simulink model "Discrete_LADRC_Control_Simulation"  (R2025a)
settings: Solver=VariableStepAuto  StartTime=0.0  StopTime=0.3  RelTol=1e-3
libraries: powerlib_extras x1
settings Model: Creator=星必尘Sguan  LastModifiedBy=星必尘Sguan
settings SFSimCC: SimCustomHeaderCode="#include \"Sguan_Ladrc.h\""  SimCustomInitializer=Sguan_Init();  SimUserSources=Sguan_Ladrc.c

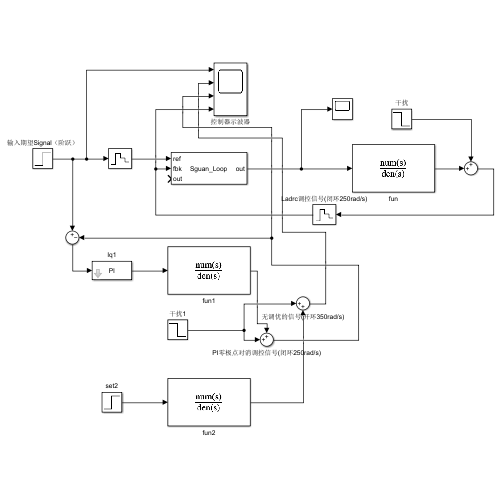
[thumbnail: Simulink's stored preview of the top-level diagram]
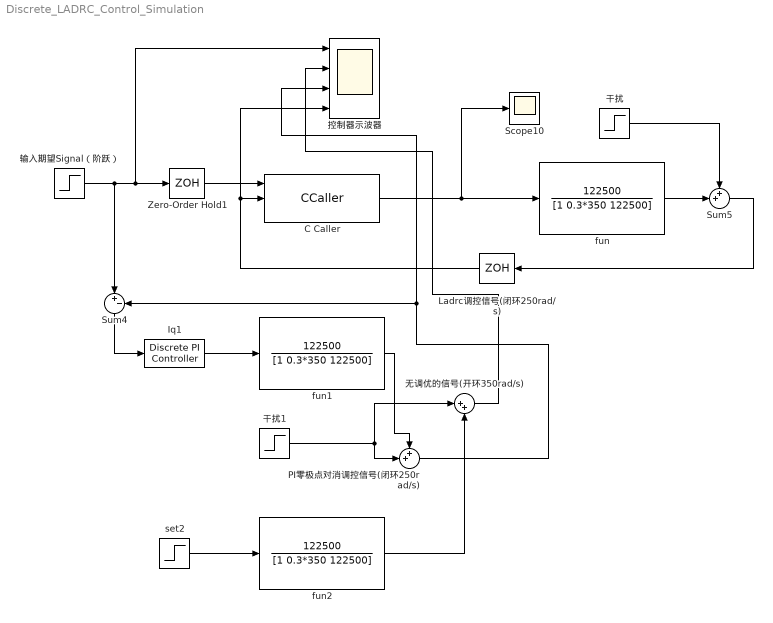
== system Discrete_LADRC_Control_Simulation ==
  C Caller : CCaller  FunctionName=Sguan_Loop  PortSpecificationStruct="%)30     .    8 4   8    (     @         %    \"     ,    !     0         %  0 \"0    $    _    07)G3F%M90  4&]R=$YA;64 4V-O<&4     26YD97@     5'EP90      4VEZ90      27-';&]B86P   X    P    !@    @    $          4    (     0    ,    !         !   P!R968 #@   #     &    \"     0         !0    @    !     P    $         $  # ')E9@ .    .     8    (    !          %    \"     $    %     0         0    !0   $EN<'5T    #@   #@    &    \"     8         !0    @    !     0    $         \"0    @               X    X    !@    @    $          4    (     0    8    !         !     &    9&]U8FQE   .    ,     8    (    !          %    \"     $    !     0         0  $ ,0    X    P    !@    @    ) @        4    (     0    $    !          (  0      #@   #     &    \"     0         !0    @    !     P    $         $  # &9B:P .    ,     8    (    !          %    \"     $    #     0         0  , 9F)K  X    X    !@    @    $          4    (     0    4    !         !     %    26YP=70    .    .     8    (    !@         %    \"     $    !     0         )    \"            / _#@   #@    &    \"     0         !0    @    !    !@    $         $     8   !D;W5B;&4   X    P    !@    @    $          4    (     0    $    !         !   0 Q    #@   #     &    \"     D\"        !0    @    !     0    $          @ !       .    ,     8    (    !          %    \"     $    #     0         0  , ;W5T  X    P    !@    @    $          4    (     0    ,    !         !   P!O=70 #@   $     &    \"     0         !0    @    !    \"P    $         $     L   !);G!U=$]U='!U=       #@   #@    &    \"     8         !0    @    !     0    $         \"0    @             0 X    X    !@    @    $          4    (     0    8    !         !     &    9&]U8FQE   .    ,     8    (    !          %    \"     $    \"     0         0  ( +3$   X    P    !@    @    ) @        4    (     0    $    !          (  0"  SampleTime=0.0005
  Iq1 : powerlib_extras/Discrete  Control Blocks/Discrete PI Controller  Kp=0.5  Ki=50  Par_Limits=[1200*0.9*sqrt(1/3) -1200*0.9*sqrt(1/3)]  Init=0  Ts=5e-4
  Ladrc调控信号(闭环250rad/s) : ZeroOrderHold  SampleTime=0.0005
  PI零极点对消调控信号(闭环250rad/s) : Sum  Inputs=++|
  Scope10 : Scope
      settings: ActiveDisplayYMinimum=-226.95199850252726  ActiveDisplayYMaximum=664.214721107104  DataLoggingVariableName=ScopeData10
  Sum4 : Sum  Inputs=|+-
  Sum5 : Sum  Inputs=++|
  Zero-Order Hold1 : ZeroOrderHold  SampleTime=0.0005
  fun : TransferFcn  Numerator=[122500]  Denominator=[1 0.3*350 122500]
  fun1 : TransferFcn  Numerator=[122500]  Denominator=[1 0.3*350 122500]
  fun2 : TransferFcn  Numerator=[122500]  Denominator=[1 0.3*350 122500]
  set2 : Step  Time=0.05  After=500  SampleTime=0
  干扰 : Step  Time=0.2  Before=-20  After=-50  SampleTime=0
  干扰1 : Step  Time=0.2  Before=-20  After=-50  SampleTime=0
  控制器示波器 : Scope  NumInputPorts=4
      settings: ActiveDisplayYMinimum=-111.30445031185839  ActiveDisplayYMaximum=901.74005280672577  DataLoggingVariableName=ScopeData9
  无调优的信号(开环350rad/s) : Sum  Inputs=|++
  输入期望Signal（阶跃） : Step  Time=0.05  After=500  SampleTime=0
  wires:
  Sum4/1 -> Iq1/1
  无调优的信号(开环350rad/s)/1 -> 控制器示波器/2
  fun/1 -> Sum5/2
  PI零极点对消调控信号(闭环250rad/s)/1 -> Sum4/2, 控制器示波器/3
  fun2/1 -> 无调优的信号(开环350rad/s)/2
  Iq1/1 -> fun1/1
  干扰/1 -> Sum5/1
  Sum5/1 -> Ladrc调控信号(闭环250rad/s)/1
  输入期望Signal（阶跃）/1 -> Sum4/1, Zero-Order Hold1/1, 控制器示波器/1
  干扰1/1 -> 无调优的信号(开环350rad/s)/1, PI零极点对消调控信号(闭环250rad/s)/2
  set2/1 -> fun2/1
  Zero-Order Hold1/1 -> C Caller/1
  fun1/1 -> PI零极点对消调控信号(闭环250rad/s)/1
  Ladrc调控信号(闭环250rad/s)/1 -> 控制器示波器/4, C Caller/2
  C Caller/1 -> Scope10/1, fun/1
